simulink library "LIB_CycleControl"  (R2018b)
settings: Solver=VariableStepAuto  StartTime=0.0  StopTime=10.0  RelTol=1e-3
undefined symbols (not defined in the file or in its folder): eActuators, eRespiratorStates, NActuatorActive, nBlowerCmdInit, nBlowerCmdMax, nBlowerCmdMin, nBlowerDecHigh, nBlowerDecMedium, nBlowerIncHigh, nBlowerIncLow, nBlowerIncMedium, NBlowerSpeedIncCorrectionGain, NBlowerValveDerivativeGain, NBlowerValveIntegralGain, NBlowerValveIntegralHighGain, NBlowerValvePropGain, NCyclePerMinMax, NCyclePerMinMin, NMaxPressureSample, NPatientValveDerivativeGain, NPatientValveIntegralGain, NPatientValveIntegralHighGain, NPatientValvePropGain, pBlowerValveOutletOffset, pDiffMaxThdForPlateauPlausibility, pDiffThdForBlowerValveControlActivation, pDiffThdForPatientValveControlActivation, pErrorPlausibilityThd, pErrorThdForHighBlowerDec, pStaticErrorThdForHighBlowerInc, rPIDIntegralMaxTermForBlowerValve, rPIDIntegralMaxTermForPatientValve, rPIDIntegralMinTermForBlowerValve, rPIDIntegralMinTermForPatientValve, tBlowerValveOpen, tDelayBeforeRespiratorCycleStart, tDelayForRespiratorStop, tPatientValveOpen, tPhase1Ofs, tStopInhalationPhase1Min
libraries: simulink x62, simulink_need_slupdate x4, simulink_extras x3
(part 4 of 4)

== system LIB_CycleControl/Cycle Control/Cycle Control Wrapper/Cycle pController/ValvePosition_Target/Inhalation/Blower Valve Control/PID Blower Valve/Integral Gain/Init ==
  rBlowerValveCmdPrev [%] : Inport
  rBlowerValveDerivative [%] : Inport  Port=2
  rBlowerValveProp [%] : Inport  Port=3
  Enable : EnablePort
  Sum2 : Sum  Inputs=+--
  Init : Outport
  wires:
  rBlowerValveDerivative [%]/1 -> Sum2/3
  Sum2/1 -> Init/1
  rBlowerValveCmdPrev [%]/1 -> Sum2/1
  rBlowerValveProp [%]/1 -> Sum2/2

== system LIB_CycleControl/Cycle Control/Cycle Control Wrapper/Cycle pController/ValvePosition_Target/Inhalation/Blower Valve Control/PID Blower Valve/Proportional Gain/Clip ==
  note: 0,0
  note: 0,0
  note: 0,0
  Upper : Inport
  In : Inport  Port=2
  Lower : Inport  Port=3
  Relational Operator : RelationalOperator  Operator=<  RndMeth=Nearest  InputSameDT=on
  Relational Operator1 : RelationalOperator  Operator=>  RndMeth=Nearest  InputSameDT=on
  Switch : Switch  Threshold=1  SaturateOnIntegerOverflow=on  InputSameDT=on
  Switch1 : Switch  Threshold=1  SaturateOnIntegerOverflow=on  InputSameDT=on
  Out : Outport
  wires:
  Switch1/1 -> Out/1
  Relational Operator1/1 -> Switch1/2
  Switch/1 -> Relational Operator1/1, Switch1/1
  Lower/1 -> Switch1/3, Relational Operator1/2
  Relational Operator/1 -> Switch/2
  Upper/1 -> Relational Operator/1, Switch/1
  In/1 -> Relational Operator/2, Switch/3

== system LIB_CycleControl/Cycle Control/Cycle Control Wrapper/Cycle pController/ValvePosition_Target/Exhalation/Patient Valve Control/PID Patient Valve/Clip MIn Max/Clip1/arround 0.001 ==
  In1 : Inport
  Gain : Gain  Gain=1000
  Gain1 : Gain  Gain=1/1000
  Rounding Function : Rounding  Operator=round
  Out1 : Outport
  wires:
  Gain/1 -> Rounding Function/1
  Rounding Function/1 -> Gain1/1
  Gain1/1 -> Out1/1
  In1/1 -> Gain/1

== system LIB_CycleControl/Cycle Control/Cycle Control Wrapper/Cycle pController/ValvePosition_Target/Exhalation/Patient Valve Control/PID Patient Valve/Derivative Gain/Compute Derivative/Clip ==
  note: 0,0
  note: 0,0
  note: 0,0
  Upper : Inport
  In : Inport  Port=2
  Lower : Inport  Port=3
  Relational Operator : RelationalOperator  Operator=<  RndMeth=Nearest  InputSameDT=on
  Relational Operator1 : RelationalOperator  Operator=>  RndMeth=Nearest  InputSameDT=on
  Switch : Switch  Threshold=1  SaturateOnIntegerOverflow=on  InputSameDT=on
  Switch1 : Switch  Threshold=1  SaturateOnIntegerOverflow=on  InputSameDT=on
  Out : Outport
  wires:
  Switch1/1 -> Out/1
  Relational Operator1/1 -> Switch1/2
  Switch/1 -> Relational Operator1/1, Switch1/1
  Lower/1 -> Switch1/3, Relational Operator1/2
  Relational Operator/1 -> Switch/2
  Upper/1 -> Relational Operator/1, Switch/1
  In/1 -> Relational Operator/2, Switch/3

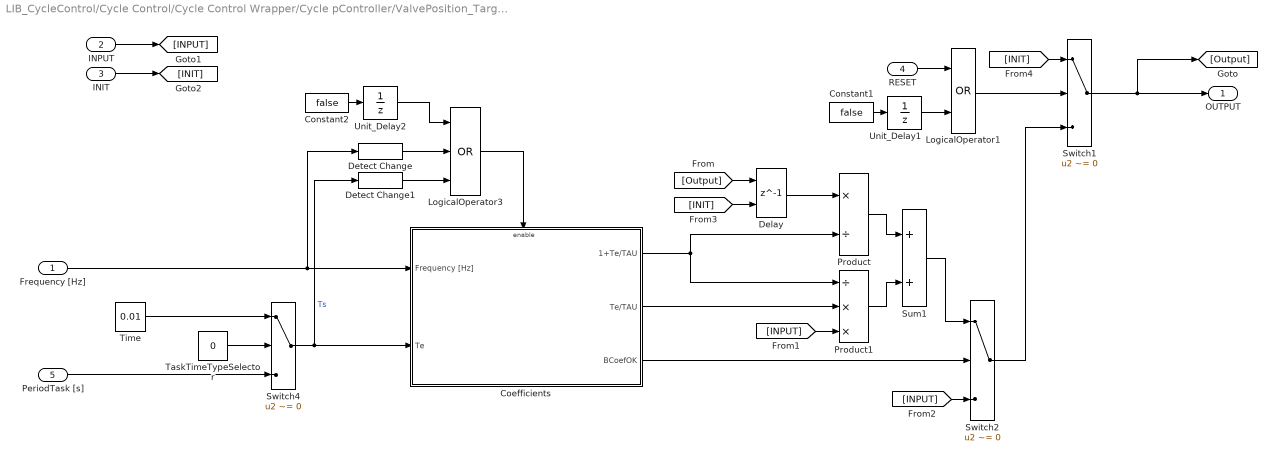
== system LIB_CycleControl/Cycle Control/Cycle Control Wrapper/Cycle pController/ValvePosition_Target/Exhalation/Patient Valve Control/PID Patient Valve/Derivative Gain/Compute Derivative/Filtre_1er_ordre_Init ==
  Frequency [Hz] : Inport  Tag=AM,In,0,1,Name,C;CMP,Port,PortWidth,SampleTime;
  INPUT : Inport  Tag=AM,In,0,1,Name,C;CMP,Port,PortWidth,SampleTime;  Port=2
  INIT : Inport  Tag=AM,In,0,1,Name,C;CMP,Port,PortWidth,SampleTime;  Port=3
  RESET : Inport  Tag=AM,In,0,1,Name,C;CMP,Port,PortWidth,SampleTime;  Port=4
  PeriodTask [s] : Inport  Tag=AM,In,0,1,Name,C;CMP,Port,PortWidth,SampleTime;  Port=5
  Coefficients : Subsystem
  Constant1 : Constant  Value=false
  Constant2 : Constant  Value=false
  Delay : Delay  DelayLength=1  InitialConditionSource=Input port  InitialCondition=0
      settings: InputPortMap=u0,p4
  Detect Change : simulink/Logic and Bit Operations/Detect Change  vinit=0  OutDataTypeStr=boolean
  Detect Change1 : simulink/Logic and Bit Operations/Detect Change  vinit=0  OutDataTypeStr=boolean
  LogicalOperator1 : Logic  Operator=OR  AllPortsSameDT=off  OutDataTypeStr=boolean
  LogicalOperator3 : Logic  Operator=OR  Inputs=3  AllPortsSameDT=off  OutDataTypeStr=boolean
  Product : Product  Inputs=*/  SaturateOnIntegerOverflow=on  RndMeth=Zero  InputSameDT=on  OutDataTypeStr=Inherit: Same as first input
  Product1 : Product  Inputs=/**  SaturateOnIntegerOverflow=on  RndMeth=Zero  InputSameDT=on  OutDataTypeStr=Inherit: Same as first input
  Sum1 : Sum  SaturateOnIntegerOverflow=on  InputSameDT=on  OutDataTypeStr=Inherit: Same as first input
  Switch1 : Switch  Tag=GEN,Threshold;AM,Switch,2,1;CMP,Threshold;  Criteria=u2 ~= 0  Threshold=0.5  SaturateOnIntegerOverflow=on  InputSameDT=on
  Switch2 : Switch  Tag=GEN,Threshold;AM,Switch,2,1;CMP,Threshold;  Criteria=u2 ~= 0  SaturateOnIntegerOverflow=on  InputSameDT=on
  Switch4 : Switch  Tag=GEN,Threshold;AM,Switch,2,1;CMP,Threshold;  Criteria=u2 ~= 0  Threshold=0.5  SaturateOnIntegerOverflow=on  InputSameDT=on
  TaskTimeTypeSelector : Constant  Value=0  OutDataTypeStr=boolean
  Time : Constant  Value=0.01  OutDataTypeStr=Inherit: Inherit via back propagation
  Unit_Delay1 : UnitDelay  InitialCondition=true  SampleTime=-1
      settings: AttributesFormatString=IC = %<X0>
  Unit_Delay2 : UnitDelay  InitialCondition=true  SampleTime=-1
      settings: AttributesFormatString=IC = %<X0>
  OUTPUT : Outport  Tag=AM,Out,1,0,Name,NC;CMP,Port,OutputWhenDisabled,InitialOutput;
  wires:
  Switch1/1 -> [Output], OUTPUT/1
  [Output] -> Delay/1
  RESET/1 -> LogicalOperator1/1
  Unit_Delay1/1 -> LogicalOperator1/2
  Delay/1 -> Product/1
  LogicalOperator1/1 -> Switch1/2
  Product1/1 -> Sum1/2
  Product/1 -> Sum1/1
  INPUT/1 -> [INPUT]
  INIT/1 -> [INIT]
  [INPUT] -> Product1/3
  [INIT] -> Delay/2
  [INIT] -> Switch1/1
  Switch2/1 -> Switch1/3
  Coefficients/1(1+Te/TAU) -> Product1/1, Product/2
  Coefficients/2(Te/TAU) -> Product1/2
  Frequency [Hz]/1 -> Coefficients/1(Frequency [Hz]), Detect Change/1
  PeriodTask [s]/1 -> Switch4/3
  Switch4/1 -> Coefficients/2(Te), Detect Change1/1  "Ts"
  Time/1 -> Switch4/1
  TaskTimeTypeSelector/1 -> Switch4/2
  LogicalOperator3/1 -> Coefficients/Enable
  Detect Change/1 -> LogicalOperator3/2
  Detect Change1/1 -> LogicalOperator3/3
  [INPUT] -> Switch2/3
  Sum1/1 -> Switch2/1
  Coefficients/3(BCoefOK) -> Switch2/2
  Constant2/1 -> Unit_Delay2/1
  Unit_Delay2/1 -> LogicalOperator3/1
  Constant1/1 -> Unit_Delay1/1

== system LIB_CycleControl/Cycle Control/Cycle Control Wrapper/Cycle pController/ValvePosition_Target/Exhalation/Patient Valve Control/PID Patient Valve/Integral Gain/Clip/arround 0.001 ==
  In1 : Inport
  Gain : Gain  Gain=1000
  Gain1 : Gain  Gain=1/1000
  Rounding Function : Rounding  Operator=round
  Out1 : Outport
  wires:
  Gain/1 -> Rounding Function/1
  Rounding Function/1 -> Gain1/1
  Gain1/1 -> Out1/1
  In1/1 -> Gain/1

== system LIB_CycleControl/Cycle Control/Cycle Control Wrapper/Cycle pController/ValvePosition_Target/Inhalation/Blower Valve Control/PID Blower Valve/Clip MIn Max/Clip1/arround 0.001 ==
  In1 : Inport
  Gain : Gain  Gain=1000
  Gain1 : Gain  Gain=1/1000
  Rounding Function : Rounding  Operator=round
  Out1 : Outport
  wires:
  Gain/1 -> Rounding Function/1
  Rounding Function/1 -> Gain1/1
  Gain1/1 -> Out1/1
  In1/1 -> Gain/1

== system LIB_CycleControl/Cycle Control/Cycle Control Wrapper/Cycle pController/ValvePosition_Target/Inhalation/Blower Valve Control/PID Blower Valve/Derivative Gain/Compute Derivative/Clip ==
  note: 0,0
  note: 0,0
  note: 0,0
  Upper : Inport
  In : Inport  Port=2
  Lower : Inport  Port=3
  Relational Operator : RelationalOperator  Operator=<  RndMeth=Nearest  InputSameDT=on
  Relational Operator1 : RelationalOperator  Operator=>  RndMeth=Nearest  InputSameDT=on
  Switch : Switch  Threshold=1  SaturateOnIntegerOverflow=on  InputSameDT=on
  Switch1 : Switch  Threshold=1  SaturateOnIntegerOverflow=on  InputSameDT=on
  Out : Outport
  wires:
  Switch1/1 -> Out/1
  Relational Operator1/1 -> Switch1/2
  Switch/1 -> Relational Operator1/1, Switch1/1
  Lower/1 -> Switch1/3, Relational Operator1/2
  Relational Operator/1 -> Switch/2
  Upper/1 -> Relational Operator/1, Switch/1
  In/1 -> Relational Operator/2, Switch/3

== system LIB_CycleControl/Cycle Control/Cycle Control Wrapper/Cycle pController/ValvePosition_Target/Inhalation/Blower Valve Control/PID Blower Valve/Derivative Gain/Compute Derivative/Filtre_1er_ordre_Init ==
  Frequency [Hz] : Inport  Tag=AM,In,0,1,Name,C;CMP,Port,PortWidth,SampleTime;
  INPUT : Inport  Tag=AM,In,0,1,Name,C;CMP,Port,PortWidth,SampleTime;  Port=2
  INIT : Inport  Tag=AM,In,0,1,Name,C;CMP,Port,PortWidth,SampleTime;  Port=3
  RESET : Inport  Tag=AM,In,0,1,Name,C;CMP,Port,PortWidth,SampleTime;  Port=4
  PeriodTask [s] : Inport  Tag=AM,In,0,1,Name,C;CMP,Port,PortWidth,SampleTime;  Port=5
  Coefficients : Subsystem
  Constant1 : Constant  Value=false
  Constant2 : Constant  Value=false
  Delay : Delay  DelayLength=1  InitialConditionSource=Input port  InitialCondition=0
      settings: InputPortMap=u0,p4
  Detect Change : simulink/Logic and Bit Operations/Detect Change  vinit=0  OutDataTypeStr=boolean
  Detect Change1 : simulink/Logic and Bit Operations/Detect Change  vinit=0  OutDataTypeStr=boolean
  LogicalOperator1 : Logic  Operator=OR  AllPortsSameDT=off  OutDataTypeStr=boolean
  LogicalOperator3 : Logic  Operator=OR  Inputs=3  AllPortsSameDT=off  OutDataTypeStr=boolean
  Product : Product  Inputs=*/  SaturateOnIntegerOverflow=on  RndMeth=Zero  InputSameDT=on  OutDataTypeStr=Inherit: Same as first input
  Product1 : Product  Inputs=/**  SaturateOnIntegerOverflow=on  RndMeth=Zero  InputSameDT=on  OutDataTypeStr=Inherit: Same as first input
  Sum1 : Sum  SaturateOnIntegerOverflow=on  InputSameDT=on  OutDataTypeStr=Inherit: Same as first input
  Switch1 : Switch  Tag=GEN,Threshold;AM,Switch,2,1;CMP,Threshold;  Criteria=u2 ~= 0  Threshold=0.5  SaturateOnIntegerOverflow=on  InputSameDT=on
  Switch2 : Switch  Tag=GEN,Threshold;AM,Switch,2,1;CMP,Threshold;  Criteria=u2 ~= 0  SaturateOnIntegerOverflow=on  InputSameDT=on
  Switch4 : Switch  Tag=GEN,Threshold;AM,Switch,2,1;CMP,Threshold;  Criteria=u2 ~= 0  Threshold=0.5  SaturateOnIntegerOverflow=on  InputSameDT=on
  TaskTimeTypeSelector : Constant  Value=0  OutDataTypeStr=boolean
  Time : Constant  Value=0.01  OutDataTypeStr=Inherit: Inherit via back propagation
  Unit_Delay1 : UnitDelay  InitialCondition=true  SampleTime=-1
      settings: AttributesFormatString=IC = %<X0>
  Unit_Delay2 : UnitDelay  InitialCondition=true  SampleTime=-1
      settings: AttributesFormatString=IC = %<X0>
  OUTPUT : Outport  Tag=AM,Out,1,0,Name,NC;CMP,Port,OutputWhenDisabled,InitialOutput;
  wires:
  Switch1/1 -> [Output], OUTPUT/1
  [Output] -> Delay/1
  RESET/1 -> LogicalOperator1/1
  Unit_Delay1/1 -> LogicalOperator1/2
  Delay/1 -> Product/1
  LogicalOperator1/1 -> Switch1/2
  Product1/1 -> Sum1/2
  Product/1 -> Sum1/1
  INPUT/1 -> [INPUT]
  INIT/1 -> [INIT]
  [INPUT] -> Product1/3
  [INIT] -> Delay/2
  [INIT] -> Switch1/1
  Switch2/1 -> Switch1/3
  Coefficients/1(1+Te/TAU) -> Product1/1, Product/2
  Coefficients/2(Te/TAU) -> Product1/2
  Frequency [Hz]/1 -> Coefficients/1(Frequency [Hz]), Detect Change/1
  PeriodTask [s]/1 -> Switch4/3
  Switch4/1 -> Coefficients/2(Te), Detect Change1/1  "Ts"
  Time/1 -> Switch4/1
  TaskTimeTypeSelector/1 -> Switch4/2
  LogicalOperator3/1 -> Coefficients/Enable
  Detect Change/1 -> LogicalOperator3/2
  Detect Change1/1 -> LogicalOperator3/3
  [INPUT] -> Switch2/3
  Sum1/1 -> Switch2/1
  Coefficients/3(BCoefOK) -> Switch2/2
  Constant2/1 -> Unit_Delay2/1
  Unit_Delay2/1 -> LogicalOperator3/1
  Constant1/1 -> Unit_Delay1/1

== system LIB_CycleControl/Cycle Control/Cycle Control Wrapper/Cycle pController/ValvePosition_Target/Inhalation/Blower Valve Control/PID Blower Valve/Integral Gain/Clip/arround 0.001 ==
  In1 : Inport
  Gain : Gain  Gain=1000
  Gain1 : Gain  Gain=1/1000
  Rounding Function : Rounding  Operator=round
  Out1 : Outport
  wires:
  Gain/1 -> Rounding Function/1
  Rounding Function/1 -> Gain1/1
  Gain1/1 -> Out1/1
  In1/1 -> Gain/1

== system LIB_CycleControl/Cycle Control/Cycle Control Wrapper/Cycle pController/ValvePosition_Target/Exhalation/Patient Valve Control/PID Patient Valve/Derivative Gain/Compute Derivative/Filtre_1er_ordre_Init/Coefficients ==
  note: Shannon
  note: Te/Tau = Te*f*2Pi
  Frequency [Hz] : Inport
  Te : Inport  Port=2
  Enable : EnablePort
  0 : Constant  Value=1e-15  OutDataTypeStr=Inherit: Inherit via back propagation
  1 : Constant  Value=0.5  OutDataTypeStr=Inherit: Inherit via back propagation
  Constant : Constant  Value=2*pi  OutDataTypeStr=Inherit: Inherit via back propagation
  Constant2 : Constant  Value=2*pi  OutDataTypeStr=Inherit: Inherit via back propagation
  Constant3 : Constant  OutDataTypeStr=Inherit: Inherit via back propagation
  Constant5 : Constant  Value=2*pi  OutDataTypeStr=Inherit: Inherit via back propagation
  DIV : Subsystem  mask(DIV){}
      mask help: This block executes a division with protection for division by 0.
      mask Display: disp('DIV')
  Data Type Conversion3 : DataTypeConversion
  FilterInputTypeSelector : Constant  Value=0  OutDataTypeStr=boolean
  Logical Operator : Logic  AllPortsSameDT=off
  Product1 : Product  Inputs=***  SaturateOnIntegerOverflow=on  RndMeth=Zero  InputSameDT=on  OutDataTypeStr=Inherit: Same as first input
  Product2 : Product  Inputs=*/  SaturateOnIntegerOverflow=on  RndMeth=Zero  InputSameDT=on  OutDataTypeStr=Inherit: Same as first input
  Relational Operator : RelationalOperator  Operator=>  RndMeth=Nearest  InputSameDT=on
  Relational Operator1 : RelationalOperator  Operator=<  RndMeth=Nearest  InputSameDT=on
  Saturation [0-2pi] : Saturate  UpperLimit=2*pi  LowerLimit=0  OutDataTypeStr=Inherit: Inherit via back propagation
  Sum3 : Sum  OutDataTypeStr=Inherit: Inherit via back propagation  RndMeth=Zero  InputSameDT=on
  Switch4 : Switch  Tag=GEN,Threshold;AM,Switch,2,1;CMP,Threshold;  Criteria=u2 ~= 0  Threshold=0.5  SaturateOnIntegerOverflow=on  InputSameDT=on
  1+Te/TAU : Outport
  Te/TAU : Outport  Port=2
  BCoefOK : Outport  Port=3
  wires:
  Constant/1 -> DIV/3(DFLT)
  Sum3/1 -> 1+Te/TAU/1
  Constant3/1 -> Sum3/1
  Constant2/1 -> Product2/2
  Frequency [Hz]/1 -> Product1/1, DIV/1(DENOM)
  Te/1 -> Product1/2, DIV/2(NUM)
  Constant5/1 -> Product1/3
  DIV/1(RESULT) -> Switch4/1
  Product1/1 -> Switch4/3
  Switch4/1 -> Saturation [0-2pi]/1
  FilterInputTypeSelector/1 -> Switch4/2
  Product2/1 -> Relational Operator1/1
  Relational Operator1/1 -> Logical Operator/2
  Relational Operator/1 -> Logical Operator/1
  1/1 -> Relational Operator1/2
  Saturation [0-2pi]/1 -> Te/TAU/1, Product2/1, Relational Operator/1, Sum3/2
  0/1 -> Data Type Conversion3/1
  Data Type Conversion3/1 -> Relational Operator/2
  Logical Operator/1 -> BCoefOK/1

== system LIB_CycleControl/Cycle Control/Cycle Control Wrapper/Cycle pController/ValvePosition_Target/Inhalation/Blower Valve Control/PID Blower Valve/Derivative Gain/Compute Derivative/Filtre_1er_ordre_Init/Coefficients ==
  note: Shannon
  note: Te/Tau = Te*f*2Pi
  Frequency [Hz] : Inport
  Te : Inport  Port=2
  Enable : EnablePort
  0 : Constant  Value=1e-15  OutDataTypeStr=Inherit: Inherit via back propagation
  1 : Constant  Value=0.5  OutDataTypeStr=Inherit: Inherit via back propagation
  Constant : Constant  Value=2*pi  OutDataTypeStr=Inherit: Inherit via back propagation
  Constant2 : Constant  Value=2*pi  OutDataTypeStr=Inherit: Inherit via back propagation
  Constant3 : Constant  OutDataTypeStr=Inherit: Inherit via back propagation
  Constant5 : Constant  Value=2*pi  OutDataTypeStr=Inherit: Inherit via back propagation
  DIV : Subsystem  mask(DIV){}
      mask help: This block executes a division with protection for division by 0.
      mask Display: disp('DIV')
  Data Type Conversion3 : DataTypeConversion
  FilterInputTypeSelector : Constant  Value=0  OutDataTypeStr=boolean
  Logical Operator : Logic  AllPortsSameDT=off
  Product1 : Product  Inputs=***  SaturateOnIntegerOverflow=on  RndMeth=Zero  InputSameDT=on  OutDataTypeStr=Inherit: Same as first input
  Product2 : Product  Inputs=*/  SaturateOnIntegerOverflow=on  RndMeth=Zero  InputSameDT=on  OutDataTypeStr=Inherit: Same as first input
  Relational Operator : RelationalOperator  Operator=>  RndMeth=Nearest  InputSameDT=on
  Relational Operator1 : RelationalOperator  Operator=<  RndMeth=Nearest  InputSameDT=on
  Saturation [0-2pi] : Saturate  UpperLimit=2*pi  LowerLimit=0  OutDataTypeStr=Inherit: Inherit via back propagation
  Sum3 : Sum  OutDataTypeStr=Inherit: Inherit via back propagation  RndMeth=Zero  InputSameDT=on
  Switch4 : Switch  Tag=GEN,Threshold;AM,Switch,2,1;CMP,Threshold;  Criteria=u2 ~= 0  Threshold=0.5  SaturateOnIntegerOverflow=on  InputSameDT=on
  1+Te/TAU : Outport
  Te/TAU : Outport  Port=2
  BCoefOK : Outport  Port=3
  wires:
  Constant/1 -> DIV/3(DFLT)
  Sum3/1 -> 1+Te/TAU/1
  Constant3/1 -> Sum3/1
  Constant2/1 -> Product2/2
  Frequency [Hz]/1 -> Product1/1, DIV/1(DENOM)
  Te/1 -> Product1/2, DIV/2(NUM)
  Constant5/1 -> Product1/3
  DIV/1(RESULT) -> Switch4/1
  Product1/1 -> Switch4/3
  Switch4/1 -> Saturation [0-2pi]/1
  FilterInputTypeSelector/1 -> Switch4/2
  Product2/1 -> Relational Operator1/1
  Relational Operator1/1 -> Logical Operator/2
  Relational Operator/1 -> Logical Operator/1
  1/1 -> Relational Operator1/2
  Saturation [0-2pi]/1 -> Te/TAU/1, Product2/1, Relational Operator/1, Sum3/2
  0/1 -> Data Type Conversion3/1
  Data Type Conversion3/1 -> Relational Operator/2
  Logical Operator/1 -> BCoefOK/1

== system LIB_CycleControl/Cycle Control/Cycle Control Wrapper/Cycle pController/ValvePosition_Target/Exhalation/Patient Valve Control/PID Patient Valve/Derivative Gain/Compute Derivative/Filtre_1er_ordre_Init/Coefficients/DIV ==
  DENOM : Inport
  NUM : Inport  Port=2
  DFLT : Inport  Port=3
  Action_Else : Subsystem  TreatAsAtomicUnit=on
  Action_If : Subsystem  TreatAsAtomicUnit=on
  If : If  IfExpression=u1 ~= 0
  Merge : Merge
  RESULT : Outport
  wires:
  Merge/1 -> RESULT/1
  Action_Else/1(RESULT) -> Merge/2
  Action_If/1(RESULT) -> Merge/1
  If/2 -> Action_Else/Action
  DFLT/1 -> Action_Else/1(DFLT)
  DENOM/1 -> If/1, Action_If/2(DENOM)
  NUM/1 -> Action_If/1(NUM)
  If/1 -> Action_If/Action

== system LIB_CycleControl/Cycle Control/Cycle Control Wrapper/Cycle pController/ValvePosition_Target/Inhalation/Blower Valve Control/PID Blower Valve/Derivative Gain/Compute Derivative/Filtre_1er_ordre_Init/Coefficients/DIV ==
  DENOM : Inport
  NUM : Inport  Port=2
  DFLT : Inport  Port=3
  Action_Else : Subsystem  TreatAsAtomicUnit=on
  Action_If : Subsystem  TreatAsAtomicUnit=on
  If : If  IfExpression=u1 ~= 0
  Merge : Merge
  RESULT : Outport
  wires:
  Merge/1 -> RESULT/1
  Action_Else/1(RESULT) -> Merge/2
  Action_If/1(RESULT) -> Merge/1
  If/2 -> Action_Else/Action
  DFLT/1 -> Action_Else/1(DFLT)
  DENOM/1 -> If/1, Action_If/2(DENOM)
  NUM/1 -> Action_If/1(NUM)
  If/1 -> Action_If/Action

== system LIB_CycleControl/Cycle Control/Cycle Control Wrapper/Cycle pController/ValvePosition_Target/Exhalation/Patient Valve Control/PID Patient Valve/Derivative Gain/Compute Derivative/Filtre_1er_ordre_Init/Coefficients/DIV/Action_Else ==
  DFLT : Inport
  Action Port : ActionPort
  Signal Conversion : SignalConversion  OverrideOpt=off
  RESULT : Outport
  wires:
  Signal Conversion/1 -> RESULT/1
  DFLT/1 -> Signal Conversion/1

== system LIB_CycleControl/Cycle Control/Cycle Control Wrapper/Cycle pController/ValvePosition_Target/Exhalation/Patient Valve Control/PID Patient Valve/Derivative Gain/Compute Derivative/Filtre_1er_ordre_Init/Coefficients/DIV/Action_If ==
  NUM : Inport
  DENOM : Inport  Port=2
  Action Port : ActionPort
  Ideal gas law2 : Product  Inputs=*/
  RESULT : Outport
  wires:
  DENOM/1 -> Ideal gas law2/2
  Ideal gas law2/1 -> RESULT/1
  NUM/1 -> Ideal gas law2/1

== system LIB_CycleControl/Cycle Control/Cycle Control Wrapper/Cycle pController/ValvePosition_Target/Inhalation/Blower Valve Control/PID Blower Valve/Derivative Gain/Compute Derivative/Filtre_1er_ordre_Init/Coefficients/DIV/Action_Else ==
  DFLT : Inport
  Action Port : ActionPort
  Signal Conversion : SignalConversion  OverrideOpt=off
  RESULT : Outport
  wires:
  Signal Conversion/1 -> RESULT/1
  DFLT/1 -> Signal Conversion/1

== system LIB_CycleControl/Cycle Control/Cycle Control Wrapper/Cycle pController/ValvePosition_Target/Inhalation/Blower Valve Control/PID Blower Valve/Derivative Gain/Compute Derivative/Filtre_1er_ordre_Init/Coefficients/DIV/Action_If ==
  NUM : Inport
  DENOM : Inport  Port=2
  Action Port : ActionPort
  Ideal gas law2 : Product  Inputs=*/
  RESULT : Outport
  wires:
  DENOM/1 -> Ideal gas law2/2
  Ideal gas law2/1 -> RESULT/1
  NUM/1 -> Ideal gas law2/1

== stateflow chart LIB_CycleControl/Cycle Control/Cycle Control Wrapper/Cycle pController/Cycle Manager/Respiratory Cycle Management ==
  state CYCLE_ACTIVE
    entry: NCycle=0;
    tCycle=tSample;
    during: tCycle=tCycle+tSample;
    state START
      entry :
      BRespiratorCycleStopped=false;
      NRespiratorCycleStatus...
      =eRespiratorStates.NRespiratorStart;
    state INHALATION
      entry: fCallCycleComputation;
      tCycle=tSample;
      state PRESSURE_RISE
        entry: NRespiratorCycleStatus...
        =eRespiratorStates.NRespiratorInInhalationPhase1;
        tStopInhalationPhase1=0;
      state PRESSURE_HOLD
        entry: NRespiratorCycleStatus...
        =eRespiratorStates.NRespiratorInInhalationPhase2;
      (default) -> PRESSURE_RISE
      PRESSURE_RISE -> PRESSURE_HOLD : [(tCycle-tSample)>0.8*tInhalationMaxDuration...
          | ||pBlowerValveOutlet>pBlowerValveOutletPlateauTargetApplied-pBlowerValveOutletOffset]
          | {tStopInhalationPhase1=tCycle-tSample;}
    state EXHALATION
      entry: NRespiratorCycleStatus...
      =eRespiratorStates.NRespiratorInExhalation;
    (default) -> START
    START -> INHALATION : [tCycle>tDelayBeforeRespiratorCycleStart+tSample/2]
        | {NCycle=1;}
    (junction 67) -> INHALATION [order 1] : [NCycle<65535]{NCycle=NCycle+1;}
    (junction 67) -> INHALATION [order 2] : {NCycle=1;}
    INHALATION -> EXHALATION : [tCycle>tInhalationMaxDuration+tSample/2]
    EXHALATION -> (junction 67) : [tCycle>tCycleMaxDuration+tSample/2]
  state NOCYCLE_ACTIVE
    entry :
    tCycle=0;
    NRespiratorCycleStatus...
    =eRespiratorStates.NRespiratorStop;
    state RespiratorStopping
      (default) -> (junction 124)
      (junction 124) -> (junction 99) : [~BRespiratorCycleStopped]
      (junction 99) -> (junction 102) [order 1] : [tCycle<tDelayForRespiratorStop-tSample/2]
      (junction 99) -> (junction 107) [order 2] : {BRespiratorCycleStopped=true}
      (junction 102) -> (junction 109) : {tCycle=tCycle+tSample;}
      (junction 107) -> (junction 109)
    (default) -> RespiratorStopping
    RespiratorStopping -> RespiratorStopping
  (default) -> (junction 117)
  (junction 117) -> CYCLE_ACTIVE [order 1] : [BRespiratorCycleRunRequest...
      | &&~BRespiratorCycleStopRequest]
  (junction 117) -> NOCYCLE_ACTIVE [order 2] : {BRespiratorCycleStopped=true;}
  CYCLE_ACTIVE -> NOCYCLE_ACTIVE : [BRespiratorCycleStopRequest]
  NOCYCLE_ACTIVE -> CYCLE_ACTIVE : [BRespiratorCycleRunRequest...
      | &&BRespiratorCycleStopped]
  data: BRespiratorCycleRunRequest input [0..1]; BRespiratorCycleStopRequest input [0..1]; NRespiratorCycleStatus output Enum: eRespiratorStates =eRespiratorStates.NRespiratorStop; tInhalationMaxDuration input [0..65535]; tCycleMaxDuration input [0..65535]; tSample input [0..65535]; pBlowerValveOutlet input [0..2000]; pBlowerValveOutletPlateauTargetApplied input [0..2000]; tCycle output single [0..65535]; pBlowerValveOutletOffset input [0..2000]; tDelayBeforeRespiratorCycleStart input [0..65535]; NCycle output single [0..65535]; tStopInhalationPhase1 output single [0..65535]; BRespiratorCycleStopped output boolean [0..1]; tDelayForRespiratorStop input [0..65535]
  events: fCallCycleComputation output FUNCTION_CALL_EVENT
